simulink model "pd_fuzzy"  (R2019b)
settings: Solver=VariableStepAuto  StartTime=0.0  StopTime=100  RelTol=1e-3
libraries: fuzblock x1
settings Model: Creator=frederick  LastModifiedBy=frede

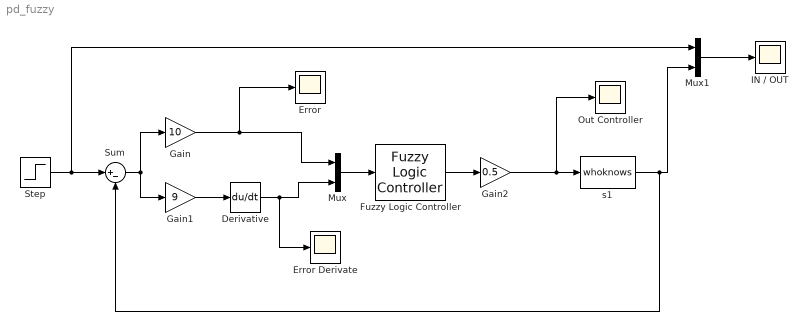
== system pd_fuzzy ==
  Derivative : Derivative
  Error : Scope
  Error Derivate : Scope
  Fuzzy Logic Controller : fuzblock/Fuzzy Logic  Controller  FIS='pd_fuzzy.fis'  OutputSampleNumber=101  DataType=double  FuzzifiedInputs=off  RuleFiringStrengths=off  RuleOutputs=off  AggregatedOutputs=off  SimulateUsing=Interpreted execution  OutOfRangeInputValueMessage=warning  NoRuleFiredMessage=warning  EmptyOutputFuzzySetMessage=warning
  Gain : Gain  Gain=10
  Gain1 : Gain  Gain=9
  Gain2 : Gain  Gain=0.5
  "IN / OUT " : Scope
  Mux : Mux  Inputs=2
  Mux1 : Mux  Inputs=2
  Out Controller : Scope
  Step : Step  SampleTime=0
  Sum : Sum  Inputs=|+-
  s1 : M-S-Function  FunctionName=whoknows  Parameters=L, P1, P2, T, R  mask{L=7, P1=1, P2=3, T=2, R=0}
      mask prompts: L "Laboratorio"; P1 "Primer digito del Puesto"; P2 "Segundo digito del Puesto"; T "Tipo de Planta"; R "Ruido"
      mask Display: disp('Sistema')
  wires:
  Mux/1 -> Fuzzy Logic Controller/1
  Fuzzy Logic Controller/1 -> Gain2/1
  Step/1 -> Mux1/1, Sum/1
  Sum/1 -> Gain/1, Gain1/1
  Derivative/1 -> Error Derivate/1, Mux/2
  Mux1/1 -> "IN / OUT "/1
  s1/1 -> Mux1/2, Sum/2
  Gain/1 -> Mux/1, Error/1
  Gain1/1 -> Derivative/1
  Gain2/1 -> Out Controller/1, s1/1
